simulink model "task3"  (R2024a)
settings: Solver=VariableStepAuto  StartTime=0.0  StopTime=15  FixedStep=1  RelTol=1e-15
settings Model: Creator=kit  LastModifiedBy=kit

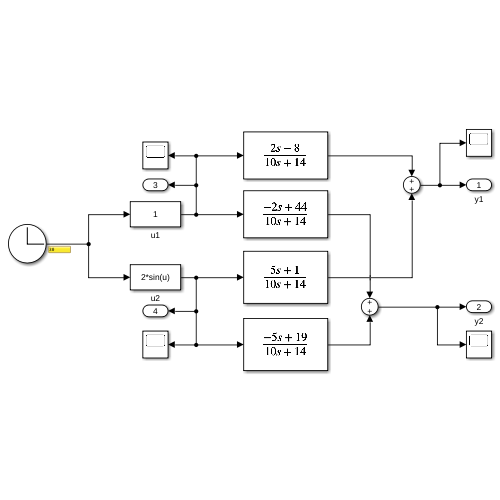
[thumbnail: Simulink's stored preview of the top-level diagram]
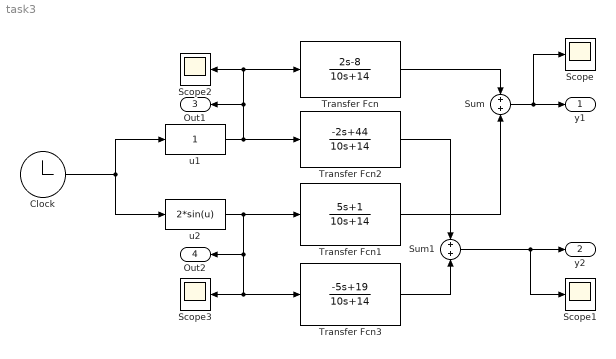
== system task3 ==
  Clock : Clock
  Scope{,1..3} (4 alike) : Scope
  Sum : Sum
  Sum1 : Sum
  Transfer Fcn : TransferFcn  Numerator=[2 -8]  Denominator=[10 14]
  Transfer Fcn1 : TransferFcn  Numerator=[5 1]  Denominator=[10 14]
  Transfer Fcn2 : TransferFcn  Numerator=[-2 44]  Denominator=[10 14]
  Transfer Fcn3 : TransferFcn  Numerator=[-5 19]  Denominator=[10 14]
  u1 : Fcn  Expr=1
  u2 : Fcn  Expr=2*sin(u)
  y1 : Outport
  y2 : Outport  Port=2
  Out1 : Outport  Port=3
  Out2 : Outport  Port=4
  wires:
  Clock/1 -> u2/1, u1/1
  u1/1 -> Out1/1, Transfer Fcn/1, Scope2/1, Transfer Fcn2/1
  u2/1 -> Transfer Fcn1/1, Transfer Fcn3/1, Scope3/1, Out2/1
  Transfer Fcn/1 -> Sum/1
  Transfer Fcn1/1 -> Sum/2
  Transfer Fcn3/1 -> Sum1/2
  Transfer Fcn2/1 -> Sum1/1
  Sum1/1 -> Scope1/1, y2/1
  Sum/1 -> Scope/1, y1/1
